simulink model "helicoptertemplate_lqi_test"  (R2021b)
settings: Solver=ode45  StartTime=0.0  StopTime=Tsim  RelTol=1e-3
InitFcn:
  | hwinit
values from neighbouring files (symbols this model uses):
  adingain = [pitchgain 1 1 1]    [hwinit.m]
  adinoffs = [pitchoffs 0 0 0]    [hwinit.m]
  h = 0.01    [LQR_LQI_init.m]
undefined symbols (not defined in the file or in its folder): DiscIntNeverNeededParam, HeliMexHandle, Kd
libraries: eeGeneralControl x1, eeLuenbergerObserver x1
settings Model: Creator=fkzhang  LastModifiedBy=rjvanderhorst
settings SolverCC: AlgebraicLoopSolver=TrustRegion
settings DataIOCC: LimitDataPoints=on  SaveFormat=Array  ReturnWorkspaceOutputs=off
settings OptimizationCC: BlockReduction=off  BooleanDataType=off  LifeSpan=inf
settings DebuggingCC: SaveWithParameterizedLinksMsg=none  UnderspecifiedInitializationDetection=Classic  MergeDetectMultiDrivingBlocksExec=none  SignalResolutionControl=TryResolveAllWithWarning  AllowSymbolicDim=off  SFUnexpectedBacktrackingDiag=warning  SFNoUnconditionalDefaultTransitionDiag=warning  SFExecutionAtInitializationDiag=none  SFMachineParentedDataDiag=warning  ArithmeticOperatorsInVariantConditions=warning
settings HardwareCC: ProdBitPerPointer=32  ProdBitPerSizeT=32  ProdBitPerPtrDiffT=32  ProdLargestAtomicFloat=None  ProdIntDivRoundTo=Undefined  ProdEndianess=Unspecified  ProdWordSize=32  ProdHWDeviceType=32-bit Generic  TargetUnknown=on
settings ModelReferenceCC: PropagateSignalLabelsOutOfModel=off
settings SFSimCC: SimUseLocalCustomCode=off  CustomCodeUndefinedFunction=UseInterfaceOnly
settings RTWCC: RTWUseLocalCustomCode=off
settings CodeAppCC: StateflowObjectComments=on
settings GRTTargetCC: TargetLangStandard=C89/C90 (ANSI)
settings ConfigComp: CovMetricSettings=dw  CovSaveCumulativeToWorkspaceVar=on  CovSaveSingleToWorkspaceVar=on  CovExternalEMLEnable=off  CovSFcnEnable=off

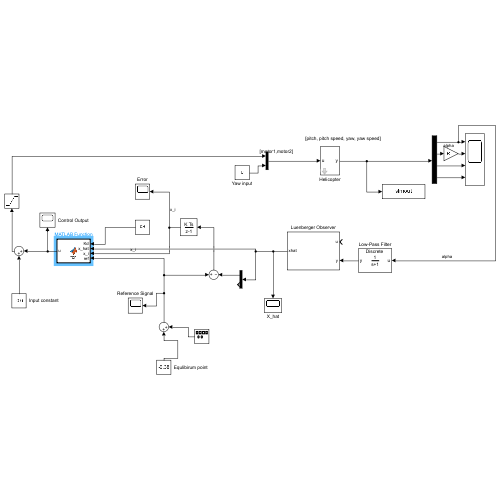
[thumbnail: Simulink's stored preview of the top-level diagram]
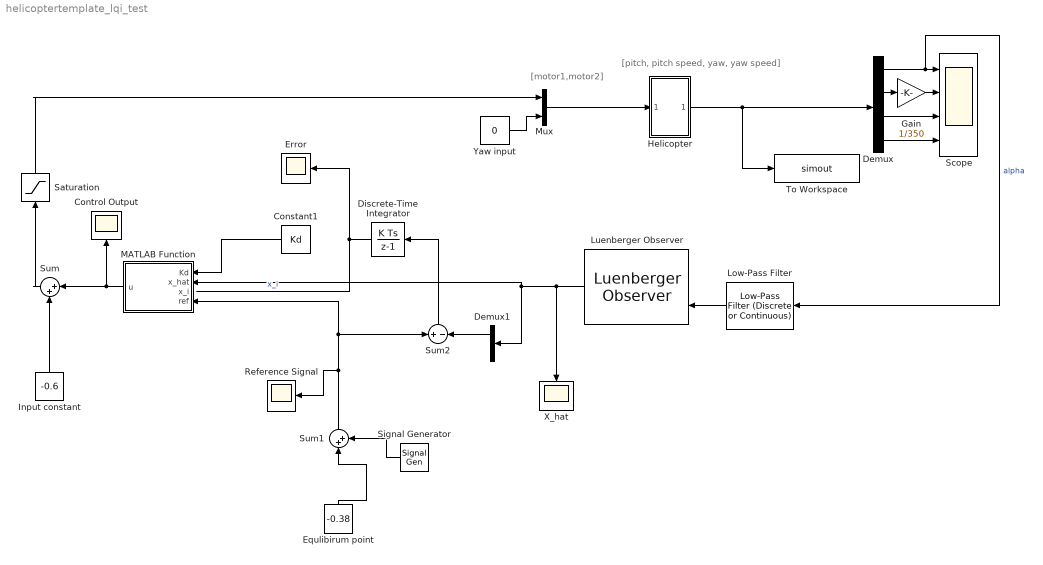
== system helicoptertemplate_lqi_test ==
  note: [pitch, pitch speed, yaw, yaw speed]
  note: [motor1,motor2]
  Constant1 : Constant  Value=Kd  LockScale=on
  Control Output : Scope
  Demux : Demux
  Demux1 : Demux  Outputs=2
  Discrete-Time Integrator : DiscreteIntegrator  SampleTime=-1  ICPrevOutput=DiscIntNeverNeededParam  ICPrevScaledInput=DiscIntNeverNeededParam
  Equlibirum point : Constant  Value=-0.38
  Error : Scope
  Gain : Gain  Gain=1/350
  Helicopter : Subsystem  mask{Ts=h}
      mask prompts: Ts "sampletime"
      mask init:
      | sf_heli_init
      mask Display:
      | port_label('input',1,'u');
      | port_label('output',1,'y');
  Input constant : Constant  Value=-0.6
  Low-Pass Filter : eeGeneralControl/Low-Pass Filter (Discrete or Continuous)  K=1  T=1  B=inf  A=-inf  init_option=Inherited from block input  x0=0  Ts=-1
  Luenberger Observer : eeLuenbergerObserver/Luenberger Observer  StateSpaceType=Discrete-time  Ad=sysd.A  Bd=sysd.B  Cd=sysd.C  Dd=sysd.D  A=1  B=1  C=1  D=1  ObserverDesign=Desired eigenvalues  Ld=2  DesiredEigenvalues=[-0.33, -0.1]  x0=[0;0]  Tsd=0.1  Ts=h
      settings: SourceProductBaseCode=PS
  MATLAB Function : MATLAB Function  TreatAsAtomicUnit=on
  Mux : Mux  Inputs=2
  Reference Signal : Scope
  Saturation : Saturate  UpperLimit=0  LowerLimit=-1
  Scope : Scope  NumInputPorts=4
  Signal Generator : SignalGenerator  Amplitude=0  Frequency=0.5  Units=rad/sec
  Sum : Sum  Inputs=|++
  Sum1 : Sum  Inputs=|++
  Sum2 : Sum  Inputs=+|-
  To Workspace : ToWorkspace  VariableName=simout  SaveFormat=Structure With Time  SampleTime=-1
  X_hat : Scope
  Yaw input : Constant  Value=0
  wires:
  Helicopter/1(Out1) -> To Workspace/1, Demux/1
  Mux/1 -> Helicopter/1(In1)
  Yaw input/1 -> Mux/2
  Demux/3 -> Scope/3
  Demux/4 -> Scope/4
  Demux/2 -> Gain/1
  Gain/1 -> Scope/2
  Demux/1 -> Low-Pass Filter/1, Scope/1  "alpha"
  Low-Pass Filter/1 -> Luenberger Observer/2
  Constant1/1 -> MATLAB Function/1(Kd)
  Input constant/1 -> Sum/2
  Sum/1 -> Saturation/1
  MATLAB Function/1(u) -> Sum/1, Control Output/1
  Saturation/1 -> Mux/1
  Equlibirum point/1 -> Sum1/1
  Sum2/1 -> Discrete-Time Integrator/1
  Discrete-Time Integrator/1 -> Error/1  "x_i"
  Luenberger Observer/1 -> Demux1/1, MATLAB Function/2(x_hat), X_hat/1
  Demux1/1 -> Sum2/2
  Signal Generator/1 -> Sum1/2
  Sum1/1 -> MATLAB Function/4(ref), Sum2/1, Reference Signal/1

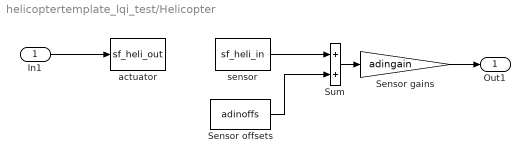
== system helicoptertemplate_lqi_test/Helicopter ==
  In1 : Inport
  Sensor gains : Gain  Gain=adingain
  Sensor offsets : Constant  Value=adinoffs
  Sum : Sum
  actuator : M-S-Function  FunctionName=sf_heli_out  Parameters=HeliMexHandle,Ts
  sensor : M-S-Function  FunctionName=sf_heli_in  Parameters=HeliMexHandle
  Out1 : Outport
  wires:
  sensor/1 -> Sum/1
  In1/1 -> actuator/1
  Sensor offsets/1 -> Sum/2
  Sum/1 -> Sensor gains/1
  Sensor gains/1 -> Out1/1

== matlab function helicoptertemplate_lqi_test/MATLAB Function ==
  data: Kd input; x_hat input; x_i input; u output; ref input
function u = fcn(Kd, x_hat, x_i, ref)
    x_ref = [ref; 0];
    error = x_hat-x_ref;
    state_vec = [error; x_i];
    u = (-Kd'*state_vec);
end
